simulink model "kundur_to_area_ps"  (R2018a)
settings: Solver=VariableStepDiscrete  StartTime=0.0  StopTime=10.0  RelTol=1e-3
libraries: powerlib x43, sps_avr x3, simulink x3, powerlib_meascontrol x1
settings Model: Creator=Bhaskar  LastModifiedBy=Bhaskar

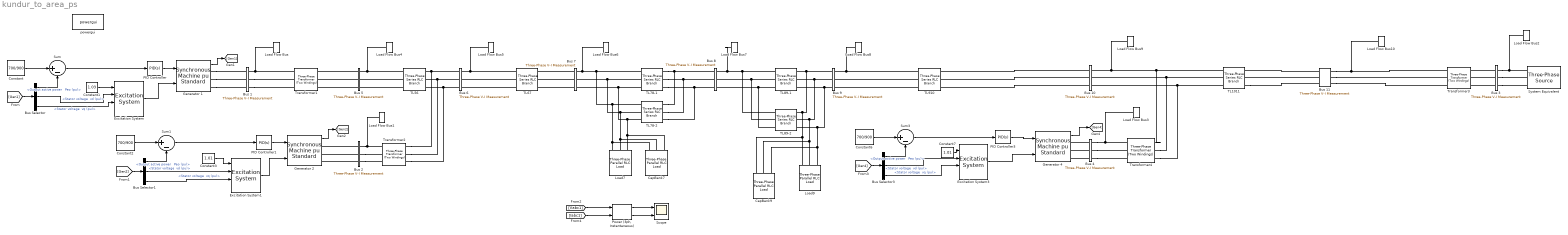
== system kundur_to_area_ps ==
  " Transformer1 " : powerlib/Elements/Three-Phase Transformer (Two Windings)  Winding1Connection=Yg  Winding2Connection=Yg  CoreType=Three single-phase transformers  SetSaturation=off  Hysteresis=off  DataFile='hysteresis'  SetInitialFlux=off  Measurements=None  UNITS=pu  NominalPower=[ 900e6 60]  Winding1=[ 20e3 0 198.944e-6 ]  Winding2="[ 230e3  0 198.944e-6]"  Rm=500  Lm=500  L0=0.5  Saturation=[ 0,0 ; 0.0024,1.2 ; 1.0,1.52 ]  InitialFluxes=[ 0.8 , -0.8 , 0.7 ]  MoreParameters=off  BreakLoop=off  DataType=off  TransfoNumber=1
  " Transformer2" : powerlib/Elements/Three-Phase Transformer (Two Windings)  Winding1Connection=Yg  Winding2Connection=Yg  CoreType=Three single-phase transformers  SetSaturation=off  Hysteresis=off  DataFile='hysteresis'  SetInitialFlux=off  Measurements=None  UNITS=pu  NominalPower=[ 900e6 60]  Winding1=[ 20e3 0 198.944e-6 ]  Winding2="[ 230e3  0 198.944e-6]"  Rm=500  Lm=500  L0=0.5  Saturation=[ 0,0 ; 0.0024,1.2 ; 1.0,1.52 ]  InitialFluxes=[ 0.8 , -0.8 , 0.7 ]  MoreParameters=off  BreakLoop=off  DataType=off  TransfoNumber=1
  " Transformer3" : powerlib/Elements/Three-Phase Transformer (Two Windings)  Winding1Connection=Yg  Winding2Connection=Yg  CoreType=Three single-phase transformers  SetSaturation=off  Hysteresis=off  DataFile='hysteresis'  SetInitialFlux=off  Measurements=None  UNITS=pu  NominalPower=[ 900e6 60]  Winding1=[ 20e3 0 198.944e-6 ]  Winding2="[ 230e3  0 198.944e-6]"  Rm=500  Lm=500  L0=0.5  Saturation=[ 0,0 ; 0.0024,1.2 ; 1.0,1.52 ]  InitialFluxes=[ 0.8 , -0.8 , 0.7 ]  MoreParameters=off  BreakLoop=off  DataType=off  TransfoNumber=1
  " Transformer4" : powerlib/Elements/Three-Phase Transformer (Two Windings)  Winding1Connection=Yg  Winding2Connection=Yg  CoreType=Three single-phase transformers  SetSaturation=off  Hysteresis=off  DataFile='hysteresis'  SetInitialFlux=off  Measurements=None  UNITS=pu  NominalPower=[ 900e6 60]  Winding1=[ 20e3 0 198.944e-6 ]  Winding2="[ 230e3  0 198.944e-6]"  Rm=500  Lm=500  L0=0.5  Saturation=[ 0,0 ; 0.0024,1.2 ; 1.0,1.52 ]  InitialFluxes=[ 0.8 , -0.8 , 0.7 ]  MoreParameters=off  BreakLoop=off  DataType=off  TransfoNumber=1
  " CapBank7" : powerlib/Elements/Three-Phase Parallel RLC Load  LConnTagsString=A|B|C  Configuration=Y (grounded)  NominalVoltage=230e3*0.8959  Vabc=[1e3 1e3 1e3]  Vabcp=[1e3 1e3 1e3]  NominalFrequency=60  UnbalancedPower=off  ActivePower=0  InductivePower=0  CapacitivePower=200e6  Pabc=[10e3 9e3 11e3]  QLabc=[100 90 110]  QCabc=[100 90 110]  Pabcp=[10e3 9e3 11e3]  QLabcp=[100 90 110]  QCabcp=[100 90 110]  Measurements=None  LoadType=constant Z
  " CapBank9" : powerlib/Elements/Three-Phase Parallel RLC Load  LConnTagsString=A|B|C  Configuration=Y (grounded)  NominalVoltage=230e3*0.9667  Vabc=[1e3 1e3 1e3]  Vabcp=[1e3 1e3 1e3]  NominalFrequency=60  UnbalancedPower=off  ActivePower=0  InductivePower=0  CapacitivePower=350e6  Pabc=[10e3 9e3 11e3]  QLabc=[100 90 110]  QCabc=[100 90 110]  Pabcp=[10e3 9e3 11e3]  QLabcp=[100 90 110]  QCabcp=[100 90 110]  Measurements=None  LoadType=constant Z
  " Load7" : powerlib/Elements/Three-Phase Parallel RLC Load  LConnTagsString=A|B|C  Configuration=Y (grounded)  NominalVoltage=230e3*0.8959  Vabc=[1e3 1e3 1e3]  Vabcp=[1e3 1e3 1e3]  NominalFrequency=60  UnbalancedPower=off  ActivePower=967e6  InductivePower=100e6  CapacitivePower=0  Pabc=[10e3 9e3 11e3]  QLabc=[100 90 110]  QCabc=[100 90 110]  Pabcp=[10e3 9e3 11e3]  QLabcp=[100 90 110]  QCabcp=[100 90 110]  Measurements=None  LoadType=constant Z
  " Load9" : powerlib/Elements/Three-Phase Parallel RLC Load  LConnTagsString=A|B|C  Configuration=Y (grounded)  NominalVoltage=230e3*0.9667  Vabc=[1e3 1e3 1e3]  Vabcp=[1e3 1e3 1e3]  NominalFrequency=60  UnbalancedPower=off  ActivePower=1767e6  InductivePower=100e6  CapacitivePower=0  Pabc=[10e3 9e3 11e3]  QLabc=[100 90 110]  QCabc=[100 90 110]  Pabcp=[10e3 9e3 11e3]  QLabcp=[100 90 110]  QCabcp=[100 90 110]  Measurements=None  LoadType=constant Z
  Bus Selector : BusSelector  OutputSignals="Output active power   Peo (pu),dq0 components.Stator voltage  vd (pu),dq0 components.Stator voltage  vq (pu)"
  Bus Selector1 : BusSelector  OutputSignals="Output active power   Peo (pu),dq0 components.Stator voltage  vd (pu),dq0 components.Stator voltage  vq (pu)"
  Bus Selector3 : BusSelector  OutputSignals="Output active power   Peo (pu),dq0 components.Stator voltage  vd (pu),dq0 components.Stator voltage  vq (pu)"
  Bus 1 : powerlib/Measurements/Three-Phase V-I Measurement  VoltageMeasurement=phase-to-ground  SetLabelV=on  LabelV=Vabc1  Vpu=off  VpuLL=off  CurrentMeasurement=yes  SetLabelI=on  LabelI=Iabc1  Ipu=off  Pbase=100e6  Vbase=500e3  OutputType=Complex  PhasorSimulation=off  PSBequivalent=0
  Bus 10 : powerlib/Measurements/Three-Phase V-I Measurement  VoltageMeasurement=phase-to-ground  SetLabelV=on  LabelV=Vabc10  Vpu=off  VpuLL=off  CurrentMeasurement=yes  SetLabelI=on  LabelI=Iabc10  Ipu=off  Pbase=100e6  Vbase=500e3  OutputType=Complex  PhasorSimulation=off  PSBequivalent=0
  Bus 11 : powerlib/Measurements/Three-Phase V-I Measurement  VoltageMeasurement=phase-to-ground  SetLabelV=on  LabelV=Vabc11  Vpu=off  VpuLL=off  CurrentMeasurement=yes  SetLabelI=on  LabelI=Iabc11  Ipu=off  Pbase=100e6  Vbase=500e3  OutputType=Complex  PhasorSimulation=off  PSBequivalent=0
  Bus 2 : powerlib/Measurements/Three-Phase V-I Measurement  VoltageMeasurement=phase-to-ground  SetLabelV=on  LabelV=Vabc2  Vpu=off  VpuLL=off  CurrentMeasurement=yes  SetLabelI=on  LabelI=Iabc2  Ipu=off  Pbase=100e6  Vbase=500e3  OutputType=Complex  PhasorSimulation=off  PSBequivalent=0
  Bus 3 : powerlib/Measurements/Three-Phase V-I Measurement  VoltageMeasurement=phase-to-ground  SetLabelV=on  LabelV=Vabc3  Vpu=off  VpuLL=off  CurrentMeasurement=yes  SetLabelI=on  LabelI=Iabc3  Ipu=off  Pbase=100e6  Vbase=500e3  OutputType=Complex  PhasorSimulation=off  PSBequivalent=0
  Bus 4 : powerlib/Measurements/Three-Phase V-I Measurement  VoltageMeasurement=phase-to-ground  SetLabelV=on  LabelV=Vabc4  Vpu=off  VpuLL=off  CurrentMeasurement=yes  SetLabelI=on  LabelI=Iabc4  Ipu=off  Pbase=100e6  Vbase=500e3  OutputType=Complex  PhasorSimulation=off  PSBequivalent=0
  Bus 5 : powerlib/Measurements/Three-Phase V-I Measurement  VoltageMeasurement=phase-to-ground  SetLabelV=on  LabelV=Vabc5  Vpu=off  VpuLL=off  CurrentMeasurement=yes  SetLabelI=on  LabelI=Iabc5  Ipu=off  Pbase=100e6  Vbase=500e3  OutputType=Complex  PhasorSimulation=off  PSBequivalent=0
  Bus 6 : powerlib/Measurements/Three-Phase V-I Measurement  VoltageMeasurement=phase-to-ground  SetLabelV=on  LabelV=Vabc6  Vpu=off  VpuLL=off  CurrentMeasurement=yes  SetLabelI=on  LabelI=Iabc6  Ipu=off  Pbase=100e6  Vbase=500e3  OutputType=Complex  PhasorSimulation=off  PSBequivalent=0
  Bus 7 : powerlib/Measurements/Three-Phase V-I Measurement  VoltageMeasurement=phase-to-ground  SetLabelV=on  LabelV=Vabc7  Vpu=off  VpuLL=off  CurrentMeasurement=yes  SetLabelI=on  LabelI=Iabc7  Ipu=off  Pbase=100e6  Vbase=500e3  OutputType=Complex  PhasorSimulation=off  PSBequivalent=0
  Bus 8 : powerlib/Measurements/Three-Phase V-I Measurement  VoltageMeasurement=phase-to-ground  SetLabelV=on  LabelV=Vabc8  Vpu=off  VpuLL=off  CurrentMeasurement=yes  SetLabelI=on  LabelI=Iabc8  Ipu=off  Pbase=100e6  Vbase=500e3  OutputType=Complex  PhasorSimulation=off  PSBequivalent=0
  Bus 9 : powerlib/Measurements/Three-Phase V-I Measurement  VoltageMeasurement=phase-to-ground  SetLabelV=on  LabelV=Vabc9  Vpu=off  VpuLL=off  CurrentMeasurement=yes  SetLabelI=on  LabelI=Iabc9  Ipu=off  Pbase=100e6  Vbase=500e3  OutputType=Complex  PhasorSimulation=off  PSBequivalent=0
  Constant : Constant  Value=700/900
  Constant1 : Constant  Value=1.03
  Constant2 : Constant  Value=700/900
  Constant3 : Constant  Value=1.01
  Constant6 : Constant  Value=700/900
  Constant7 : Constant  Value=1.01
  Excitation System : sps_avr/Excitation System  tr=0.05  reg=[ 20 0.055 ]  exc=[ 1 0 ]  tgr=[ 0 0 ]  damp=[ 0.125 1.8 ]  sat=[ 0, 0 ]  lim=[ -10 10 0 ]  v0=[0.97727 1.973]
      settings: SourceProductName=Simscape Power Systems  SourceProductBaseCode=PS
  Excitation System1 : sps_avr/Excitation System  tr=0.05  reg=[ 20 0.055 ]  exc=[ 1 0 ]  tgr=[ 0 0 ]  damp=[ 0.125 1.8 ]  sat=[ 0, 0 ]  lim=[ -10 10 0 ]  v0=[0.92904 2.0814]
      settings: SourceProductName=Simscape Power Systems  SourceProductBaseCode=PS
  Excitation System3 : sps_avr/Excitation System  tr=0.05  reg=[ 20 0.055 ]  exc=[ 1 0 ]  tgr=[ 0 0 ]  damp=[ 0.125 1.8 ]  sat=[ 0, 0 ]  lim=[ -10 10 0 ]  v0=[0.99804 1.9844]
      settings: SourceProductName=Simscape Power Systems  SourceProductBaseCode=PS
  "Generator 1 " : powerlib/Machines/Synchronous Machine pu Standard  PresetModel=No  MechanicalLoad=Mechanical power Pm  ShowDetailedParameters=on  RotorType=Round  Units=per unit standard parameters  MeasurementBus=off  NominalParameters=[900e6 20e3 60]  Reactances1=[ 1.80 0.30 0.25 1.70 0.55 0.25 0.20 ]  Reactances2=[2.24 0.17 0.12 1.02 0.13 0.08]  dAxisTimeConstants=Open-circuit  qAxisTimeConstants=Open-circuit  TimeConstants1="[ 4.4849  0.0681  0.1  ]"  TimeConstants2=[ 8.0, 0.03, 0.4, 0.05 ]  TimeConstants3="[  4.49  0.0681  0.0513  ]"  TimeConstants4=[ 8.0, 0.03, 0.3371, 0.0295 ]  TimeConstants5=[ 1.01, 0.053, 0.1 ]  TimeConstants6=[ 1.3201, 0.023, 1.0, 0.07 ]  TimeConstants7=[0.012 0.003 0.003]  TimeConstants8=[ 1.3201, 0.0231, 0.3371, 0.0295 ]  StatorResistance=0.0025  Mechanical=[6.50 0.02 1]  PolePairs=20  InitialConditions=[0 9.5032 0.823193 0.823193 0.823193 39.3665 -80.6335 159.366 1.97303]  SetSaturation=off  Saturation=[0.6404,0.7127,0.8441,0.9214,0.9956,1.082,1.19,1.316,1.457;0.7,0.7698,0.8872,0.9466,0.9969,1.046,1.1,1.151,1.201]  LoadFlowParameters=[1,0,0,0,0]  TsPowergui=0  TsBlock=-1  IterativeModel=Trapezoidal non iterative  IterativeDiscreteModel=Trapezoidal non iterative  BusType=PQ  Pref=700e6  Qref=185e6  Qmin=-inf  Qmax=inf  PLF=0  QLF=0
      settings: SourceProductName=Simscape Power Systems
  "Generator 2 " : powerlib/Machines/Synchronous Machine pu Standard  PresetModel=No  MechanicalLoad=Mechanical power Pm  ShowDetailedParameters=on  RotorType=Round  Units=per unit standard parameters  MeasurementBus=off  NominalParameters=[900e6 20e3 60]  Reactances1=[ 1.80 0.30 0.25 1.70 0.55 0.25 0.20 ]  Reactances2=[2.24 0.17 0.12 1.02 0.13 0.08]  dAxisTimeConstants=Open-circuit  qAxisTimeConstants=Open-circuit  TimeConstants1="[ 4.4849  0.0681  0.1  ]"  TimeConstants2=[ 8.0, 0.03, 0.4, 0.05 ]  TimeConstants3="[  4.49  0.0681  0.0513  ]"  TimeConstants4=[ 8.0, 0.03, 0.3371, 0.0295 ]  TimeConstants5=[ 1.01, 0.053, 0.1 ]  TimeConstants6=[ 1.3201, 0.023, 1.0, 0.07 ]  TimeConstants7=[0.012 0.003 0.003]  TimeConstants8=[ 1.3201, 0.0231, 0.3371, 0.0295 ]  StatorResistance=0.0025  Mechanical=[6.50 0.02 1]  PolePairs=20  InitialConditions=[0 -1.3462 0.883102 0.883102 0.883102 24.8213 -95.1787 144.821 2.08141]  SetSaturation=off  Saturation=[0.6404,0.7127,0.8441,0.9214,0.9956,1.082,1.19,1.316,1.457;0.7,0.7698,0.8872,0.9466,0.9969,1.046,1.1,1.151,1.201]  LoadFlowParameters=[1,0,0,0,0]  TsPowergui=0  TsBlock=-1  IterativeModel=Trapezoidal non iterative  IterativeDiscreteModel=Trapezoidal non iterative  BusType=PQ  Pref=700e6  Qref=235e6  Qmin=-inf  Qmax=inf  PLF=0  QLF=0
      settings: SourceProductName=Simscape Power Systems
  Generator 4 : powerlib/Machines/Synchronous Machine pu Standard  PresetModel=No  MechanicalLoad=Mechanical power Pm  ShowDetailedParameters=on  RotorType=Round  Units=per unit standard parameters  MeasurementBus=off  NominalParameters=[900e6 20e3 60]  Reactances1=[ 1.80 0.30 0.25 1.70 0.55 0.25 0.20 ]  Reactances2=[2.24 0.17 0.12 1.02 0.13 0.08]  dAxisTimeConstants=Open-circuit  qAxisTimeConstants=Open-circuit  TimeConstants1="[ 4.4849  0.0681  0.1  ]"  TimeConstants2=[ 8.0, 0.03, 0.4, 0.05 ]  TimeConstants3="[  4.49  0.0681  0.0513  ]"  TimeConstants4=[ 8.0, 0.03, 0.3371, 0.0295 ]  TimeConstants5=[ 1.01, 0.053, 0.1 ]  TimeConstants6=[ 1.3201, 0.023, 1.0, 0.07 ]  TimeConstants7=[0.012 0.003 0.003]  TimeConstants8=[ 1.3201, 0.0231, 0.3371, 0.0295 ]  StatorResistance=0.0025  Mechanical=[6.175 0.02 1]  PolePairs=20  InitialConditions=[0 -52.16 0.811101 0.811101 0.811101 -22.028 -142.028 97.972 1.98441]  SetSaturation=off  Saturation=[0.6404,0.7127,0.8441,0.9214,0.9956,1.082,1.19,1.316,1.457;0.7,0.7698,0.8872,0.9466,0.9969,1.046,1.1,1.151,1.201]  LoadFlowParameters=[1,0,0,0,0]  TsPowergui=0  TsBlock=-1  IterativeModel=Trapezoidal non iterative  IterativeDiscreteModel=Trapezoidal non iterative  BusType=PQ  Pref=700e6  Qref=202e6  Qmin=-inf  Qmax=inf  PLF=0  QLF=0
      settings: SourceProductName=Simscape Power Systems
  Load Flow Bus : powerlib/Measurements/Load Flow Bus  LConnTagsString=a  Phases=single  Connectors=on one side  ID=BUS_1  Vbase=20e3  Vref=1  Vangle=0  VLF=0.9773  VLFb=1  VLFc=1  angleLF=54.17  angleLFb=0  angleLFc=0
      settings: SourceProductName=Simscape Power Systems
  Load Flow Bus1 : powerlib/Measurements/Load Flow Bus  LConnTagsString=a  Phases=single  Connectors=on one side  ID=BUS_2  Vbase=20e3  Vref=1  Vangle=0  VLF=0.929  VLFb=1  VLFc=1  angleLF=43.38  angleLFb=0  angleLFc=0
      settings: SourceProductName=Simscape Power Systems
  Load Flow Bus10 : powerlib/Measurements/Load Flow Bus  LConnTagsString=a  Phases=single  Connectors=on one side  ID=BUS_11  Vbase=230e3  Vref=1  Vangle=0  VLF=1.03  VLFb=1  VLFc=1  angleLF=-0.01044  angleLFb=0  angleLFc=0
      settings: SourceProductName=Simscape Power Systems
  Load Flow Bus2 : powerlib/Measurements/Load Flow Bus  LConnTagsString=a  Phases=single  Connectors=on one side  ID=BUS_3  Vbase=20e3  Vref=1.03  Vangle=0  VLF=1.03  VLFb=1  VLFc=1  angleLF=0  angleLFb=0  angleLFc=0
      settings: SourceProductName=Simscape Power Systems
  Load Flow Bus3 : powerlib/Measurements/Load Flow Bus  LConnTagsString=a  Phases=single  Connectors=on one side  ID=BUS_4  Vbase=20e3  Vref=1  Vangle=0  VLF=0.998  VLFb=1  VLFc=1  angleLF=-5.931  angleLFb=0  angleLFc=0
      settings: SourceProductName=Simscape Power Systems
  Load Flow Bus4 : powerlib/Measurements/Load Flow Bus  LConnTagsString=a  Phases=single  Connectors=on one side  ID=BUS_5  Vbase=230e3  Vref=1  Vangle=0  VLF=0.9772  VLFb=1  VLFc=1  angleLF=54.15  angleLFb=0  angleLFc=0
      settings: SourceProductName=Simscape Power Systems
  Load Flow Bus5 : powerlib/Measurements/Load Flow Bus  LConnTagsString=a  Phases=single  Connectors=on one side  ID=BUS_6  Vbase=230e3  Vref=1  Vangle=0  VLF=0.9289  VLFb=1  VLFc=1  angleLF=43.36  angleLFb=0  angleLFc=0
      settings: SourceProductName=Simscape Power Systems
  Load Flow Bus6 : powerlib/Measurements/Load Flow Bus  LConnTagsString=a  Phases=single  Connectors=on one side  ID=BUS_7  Vbase=230e3  Vref=1  Vangle=0  VLF=0.8959  VLFb=1  VLFc=1  angleLF=33.99  angleLFb=0  angleLFc=0
      settings: SourceProductName=Simscape Power Systems
  Load Flow Bus7 : powerlib/Measurements/Load Flow Bus  LConnTagsString=a  Phases=single  Connectors=on one side  ID=BUS_8  Vbase=230e3  Vref=1  Vangle=0  VLF=0.8557  VLFb=1  VLFc=1  angleLF=9.8  angleLFb=0  angleLFc=0
      settings: SourceProductName=Simscape Power Systems
  Load Flow Bus8 : powerlib/Measurements/Load Flow Bus  LConnTagsString=a  Phases=single  Connectors=on one side  ID=BUS_9  Vbase=230e3  Vref=1  Vangle=0  VLF=0.9667  VLFb=1  VLFc=1  angleLF=-12.52  angleLFb=0  angleLFc=0
      settings: SourceProductName=Simscape Power Systems
  Load Flow Bus9 : powerlib/Measurements/Load Flow Bus  LConnTagsString=a  Phases=single  Connectors=on one side  ID=BUS_10  Vbase=230e3  Vref=1  Vangle=0  VLF=0.998  VLFb=1  VLFc=1  angleLF=-5.949  angleLFb=0  angleLFc=0
      settings: SourceProductName=Simscape Power Systems
  PID Controller : simulink/Continuous/PID Controller  Controller=PID  TimeDomain=Continuous-time  SampleTime=-1  IntegratorMethod=Forward Euler  FilterMethod=Forward Euler  Form=Parallel  UseFilter=on  ControllerParametersSource=internal  P=1  I=2  D=0.2  N=100  InitialConditionSource=internal  InitialConditionForIntegrator=0  InitialConditionForFilter=0  ExternalReset=none  LimitOutput=on  UpperSaturationLimit=0.99  LowerSaturationLimit=0.50  LinearizeAsGain=on  AntiWindupMode=none  Kb=1  TrackingMode=off  Kt=1  PParamMin=[]  PParamMax=[]  IParamMin=[]  IParamMax=[]  DParamMin=[]  DParamMax=[]  NParamMin=[]  NParamMax=[]  KbParamMin=[]  KbParamMax=[]  KtParamMin=[]  KtParamMax=[]  POutMin=[]  POutMax=[]  IOutMin=[]  IOutMax=[]  DOutMin=[]  DOutMax=[]  NOutMin=[]  NOutMax=[]  KbOutMin=[]  KbOutMax=[]  KtOutMin=[]  KtOutMax=[]  IntegratorOutMin=[]  IntegratorOutMax=[]  FilterOutMin=[]  FilterOutMax=[]  SumOutMin=[]  SumOutMax=[]  SumI1OutMin=[]  SumI1OutMax=[]  SumI2OutMin=[]  SumI2OutMax=[]  SumI3OutMin=[]  SumI3OutMax=[]  SumDOutMin=[]  SumDOutMax=[]  SaturationOutMin=[]  SaturationOutMax=[]  IntegratorContinuousStateAttributes=''  IntegratorStateMustResolveToSignalObject=off  IntegratorRTWStateStorageClass=Auto  FilterContinuousStateAttributes=''  FilterStateMustResolveToSignalObject=off  FilterRTWStateStorageClass=Auto  DifferentiatorICPrevScaledInput=0  DifferentiatorOutMin=[]  DifferentiatorOutMax=[]  FilterDiffOutCoefMin=[]  FilterDiffOutCoefMax=[]  SumDenOutMin=[]  SumDenOutMax=[]  SumNumOutMin=[]  SumNumOutMax=[]  ReciprocalOutMin=[]  ReciprocalOutMax=[]  DivideOutMin=[]  DivideOutMax=[]  TunerSelectOption=Transfer Function Based (PID Tuner App)
  PID Controller1 : simulink/Continuous/PID Controller  Controller=PID  TimeDomain=Continuous-time  SampleTime=-1  IntegratorMethod=Forward Euler  FilterMethod=Forward Euler  Form=Parallel  UseFilter=on  ControllerParametersSource=internal  P=1  I=2  D=0.2  N=100  InitialConditionSource=internal  InitialConditionForIntegrator=0  InitialConditionForFilter=0  ExternalReset=none  LimitOutput=on  UpperSaturationLimit=0.99  LowerSaturationLimit=0.50  LinearizeAsGain=on  AntiWindupMode=none  Kb=1  TrackingMode=off  Kt=1  PParamMin=[]  PParamMax=[]  IParamMin=[]  IParamMax=[]  DParamMin=[]  DParamMax=[]  NParamMin=[]  NParamMax=[]  KbParamMin=[]  KbParamMax=[]  KtParamMin=[]  KtParamMax=[]  POutMin=[]  POutMax=[]  IOutMin=[]  IOutMax=[]  DOutMin=[]  DOutMax=[]  NOutMin=[]  NOutMax=[]  KbOutMin=[]  KbOutMax=[]  KtOutMin=[]  KtOutMax=[]  IntegratorOutMin=[]  IntegratorOutMax=[]  FilterOutMin=[]  FilterOutMax=[]  SumOutMin=[]  SumOutMax=[]  SumI1OutMin=[]  SumI1OutMax=[]  SumI2OutMin=[]  SumI2OutMax=[]  SumI3OutMin=[]  SumI3OutMax=[]  SumDOutMin=[]  SumDOutMax=[]  SaturationOutMin=[]  SaturationOutMax=[]  IntegratorContinuousStateAttributes=''  IntegratorStateMustResolveToSignalObject=off  IntegratorRTWStateStorageClass=Auto  FilterContinuousStateAttributes=''  FilterStateMustResolveToSignalObject=off  FilterRTWStateStorageClass=Auto  DifferentiatorICPrevScaledInput=0  DifferentiatorOutMin=[]  DifferentiatorOutMax=[]  FilterDiffOutCoefMin=[]  FilterDiffOutCoefMax=[]  SumDenOutMin=[]  SumDenOutMax=[]  SumNumOutMin=[]  SumNumOutMax=[]  ReciprocalOutMin=[]  ReciprocalOutMax=[]  DivideOutMin=[]  DivideOutMax=[]  TunerSelectOption=Transfer Function Based (PID Tuner App)
  PID Controller3 : simulink/Continuous/PID Controller  Controller=PID  TimeDomain=Continuous-time  SampleTime=-1  IntegratorMethod=Forward Euler  FilterMethod=Forward Euler  Form=Parallel  UseFilter=on  ControllerParametersSource=internal  P=1  I=2  D=0.2  N=100  InitialConditionSource=internal  InitialConditionForIntegrator=0  InitialConditionForFilter=0  ExternalReset=none  LimitOutput=on  UpperSaturationLimit=0.99  LowerSaturationLimit=0.50  LinearizeAsGain=on  AntiWindupMode=none  Kb=1  TrackingMode=off  Kt=1  PParamMin=[]  PParamMax=[]  IParamMin=[]  IParamMax=[]  DParamMin=[]  DParamMax=[]  NParamMin=[]  NParamMax=[]  KbParamMin=[]  KbParamMax=[]  KtParamMin=[]  KtParamMax=[]  POutMin=[]  POutMax=[]  IOutMin=[]  IOutMax=[]  DOutMin=[]  DOutMax=[]  NOutMin=[]  NOutMax=[]  KbOutMin=[]  KbOutMax=[]  KtOutMin=[]  KtOutMax=[]  IntegratorOutMin=[]  IntegratorOutMax=[]  FilterOutMin=[]  FilterOutMax=[]  SumOutMin=[]  SumOutMax=[]  SumI1OutMin=[]  SumI1OutMax=[]  SumI2OutMin=[]  SumI2OutMax=[]  SumI3OutMin=[]  SumI3OutMax=[]  SumDOutMin=[]  SumDOutMax=[]  SaturationOutMin=[]  SaturationOutMax=[]  IntegratorContinuousStateAttributes=''  IntegratorStateMustResolveToSignalObject=off  IntegratorRTWStateStorageClass=Auto  FilterContinuousStateAttributes=''  FilterStateMustResolveToSignalObject=off  FilterRTWStateStorageClass=Auto  DifferentiatorICPrevScaledInput=0  DifferentiatorOutMin=[]  DifferentiatorOutMax=[]  FilterDiffOutCoefMin=[]  FilterDiffOutCoefMax=[]  SumDenOutMin=[]  SumDenOutMax=[]  SumNumOutMin=[]  SumNumOutMax=[]  ReciprocalOutMin=[]  ReciprocalOutMax=[]  DivideOutMin=[]  DivideOutMax=[]  TunerSelectOption=Transfer Function Based (PID Tuner App)
  "Power (3ph, Instantaneous)" : powerlib_meascontrol/Measurements/Power (3ph, Instantaneous)
      settings: SourceProductName=Simscape Power Systems
  Scope : Scope  NumInputPorts=2
  Sum : Sum  Inputs=|+-
  Sum1 : Sum  Inputs=|+-
  Sum3 : Sum  Inputs=|+-
  System Equivalent : powerlib/Electrical Sources/Three-Phase Source  InternalConnection=Yg  VoltagePhases=off  Voltage=(20000)*1.03  PhaseAngle=0  Voltage_phases=[25e3 25e3 25e3]/sqrt(3)  PhaseAngles_phases=[0 -120 +120]  Frequency=60  NonIdealSource=off  SpecifyImpedance=off  Resistance=0.8929  Inductance=16.58e-3  ShortCircuitLevel=100e6  BaseVoltage=25e3  XRratio=7  BusType=swing  Pref=10e3  Qref=0  Prefabc=[10e3, 10e3, 10e3]  Qrefabc=[0, 0, 0]  Qmin=-inf  Qmax=inf
  TL1011 : powerlib/Elements/Three-Phase Series RLC Branch  LConnTagsString=A|B|C  RConnTagsString=A|B|C  BranchType=RL  Resistance=1.3225  Inductance=3.508e-2  Capacitance=1e-6  Measurements=None
  "TL56 " : powerlib/Elements/Three-Phase Series RLC Branch  LConnTagsString=A|B|C  RConnTagsString=A|B|C  BranchType=RL  Resistance=1.3225  Inductance=3.508e-2  Capacitance=1e-6  Measurements=None
  TL67 : powerlib/Elements/Three-Phase Series RLC Branch  LConnTagsString=A|B|C  RConnTagsString=A|B|C  BranchType=RL  Resistance=0.529  Inductance=1.403e-2  Capacitance=1e-6  Measurements=None
  TL78-1 : powerlib/Elements/Three-Phase Series RLC Branch  LConnTagsString=A|B|C  RConnTagsString=A|B|C  BranchType=RL  Resistance=5.819  Inductance=1.544e-1  Capacitance=1e-6  Measurements=None
  TL78-2 : powerlib/Elements/Three-Phase Series RLC Branch  LConnTagsString=A|B|C  RConnTagsString=A|B|C  BranchType=RL  Resistance=5.819  Inductance=1.544e-1  Capacitance=1e-6  Measurements=None
  TL89-1 : powerlib/Elements/Three-Phase Series RLC Branch  LConnTagsString=A|B|C  RConnTagsString=A|B|C  BranchType=RL  Resistance=5.819  Inductance=1.544e-1  Capacitance=1e-6  Measurements=None
  TL89-2 : powerlib/Elements/Three-Phase Series RLC Branch  LConnTagsString=A|B|C  RConnTagsString=A|B|C  BranchType=RL  Resistance=5.819  Inductance=1.544e-1  Capacitance=1e-6  Measurements=None
  TL910 : powerlib/Elements/Three-Phase Series RLC Branch  LConnTagsString=A|B|C  RConnTagsString=A|B|C  BranchType=RL  Resistance=0.529  Inductance=1.403e-2  Capacitance=1e-6  Measurements=None
  powergui : powerlib/powergui  Priority=1  SimulationMode=Discrete  SampleTime=500e-6  frequency=60  Iterations=1000  frequencyindice=60  Pbase=100e6  ErrMax=0.0001  UnitsV=kV  UnitsW=MW  buscounter=0  FunctionMessages=off  echomessages=off  EnableUseOfTLC=off  CurrentSourceSwitches=off  DisableSnubberDevices=off  DisableRonSwitches=off  DisableVfSwitches=off  DisplayEquations=off  SolverType=Tustin/Backward Euler (TBE)  Interpol=off  ExternalGateDelay=off  methode=off  Ts=100  x0status=blocks  SPID=on  SwTol=0  HookPort=off  RestoreLinks=warning  ResistiveCurrentMeasurement=off  Frange=[0:2:500]  Ylog=off  Xlog=on  ShowGrid=off  save=off  variable=ZData  structure=0  ZoomFFT=off  StartTime=0.0  cycles=1  DisplayStyle=1  fundamental=60  FreqAxis=off  MaxFrequency=1000  frequencyindicesteady=1  RmsSteady=1  display=off
  wires:
  "Generator 1 "/1 -> [Gen1]
  [Gen1] -> Bus Selector/1
  PID Controller/1 -> "Generator 1 "/1
  Sum/1 -> PID Controller/1
  Constant/1 -> Sum/1
  Bus Selector/1 -> Sum/2  "<Output active power   Peo (pu)>"
  Constant1/1 -> Excitation System/1
  Bus Selector/2 -> Excitation System/2  "<Stator voltage  vd (pu)>"
  Bus Selector/3 -> Excitation System/3  "<Stator voltage  vq (pu)>"
  Bus Selector1/3 -> Excitation System1/3  "<Stator voltage  vq (pu)>"
  Bus Selector1/2 -> Excitation System1/2  "<Stator voltage  vd (pu)>"
  Constant3/1 -> Excitation System1/1
  Bus Selector1/1 -> Sum1/2  "<Output active power   Peo (pu)>"
  Constant2/1 -> Sum1/1
  Sum1/1 -> PID Controller1/1
  [Gen2] -> Bus Selector1/1
  Excitation System/1 -> "Generator 1 "/2
  Excitation System1/1 -> "Generator 2 "/2
  PID Controller1/1 -> "Generator 2 "/1
  "Generator 2 "/1 -> [Gen2]
  Constant7/1 -> Excitation System3/1
  Bus Selector3/1 -> Sum3/2  "<Output active power   Peo (pu)>"
  Bus Selector3/2 -> Excitation System3/2  "<Stator voltage  vd (pu)>"
  [Gen4] -> Bus Selector3/1
  Sum3/1 -> PID Controller3/1
  Generator 4/1 -> [Gen4]
  PID Controller3/1 -> Generator 4/1
  Constant6/1 -> Sum3/1
  Bus Selector3/3 -> Excitation System3/3  "<Stator voltage  vq (pu)>"
  Excitation System3/1 -> Generator 4/2
  [Vabc1] -> "Power (3ph, Instantaneous)"/1
  [Iabc1] -> "Power (3ph, Instantaneous)"/2
  "Power (3ph, Instantaneous)"/1 -> Scope/1
  "Power (3ph, Instantaneous)"/2 -> Scope/2
  connections:
  Bus 1/RConn1 -- Load Flow Bus/LConn1 -- " Transformer1 "/LConn1
  Bus 1/RConn2 -- " Transformer1 "/LConn2
  Bus 1/RConn3 -- " Transformer1 "/LConn3
  "Generator 1 "/RConn1 -- Bus 1/LConn1
  "Generator 1 "/RConn2 -- Bus 1/LConn2
  "Generator 1 "/RConn3 -- Bus 1/LConn3
  Bus 5/LConn1 -- " Transformer1 "/RConn1
  Bus 5/LConn2 -- " Transformer1 "/RConn2
  Bus 5/LConn3 -- " Transformer1 "/RConn3
  "TL56 "/LConn1 -- Load Flow Bus4/LConn1 -- Bus 5/RConn1
  "TL56 "/LConn2 -- Bus 5/RConn2
  "TL56 "/LConn3 -- Bus 5/RConn3
  Bus 6/LConn3 -- " Transformer2"/RConn3 -- "TL56 "/RConn3
  Bus 6/LConn2 -- " Transformer2"/RConn2 -- "TL56 "/RConn2
  Bus 6/LConn1 -- " Transformer2"/RConn1 -- "TL56 "/RConn1
  TL67/LConn1 -- Load Flow Bus5/LConn1 -- Bus 6/RConn1
  TL67/LConn2 -- Bus 6/RConn2
  TL67/LConn3 -- Bus 6/RConn3
  Bus 7/LConn3 -- TL67/RConn3
  Bus 7/LConn2 -- TL67/RConn2
  Bus 7/LConn1 -- TL67/RConn1
  TL78-1/LConn1 -- " CapBank7"/LConn1 -- " Load7"/LConn1 -- TL78-2/LConn1 -- Load Flow Bus6/LConn1 -- Bus 7/RConn1
  TL78-1/LConn2 -- " CapBank7"/LConn2 -- " Load7"/LConn2 -- TL78-2/LConn2 -- Bus 7/RConn2
  TL78-1/LConn3 -- " CapBank7"/LConn3 -- " Load7"/LConn3 -- TL78-2/LConn3 -- Bus 7/RConn3
  TL78-1/RConn1 -- TL78-2/RConn1 -- Bus 8/LConn1
  TL78-1/RConn2 -- TL78-2/RConn2 -- Bus 8/LConn2
  TL78-1/RConn3 -- TL78-2/RConn3 -- Bus 8/LConn3
  TL89-1/LConn1 -- TL89-2/LConn1 -- Load Flow Bus7/LConn1 -- Bus 8/RConn1
  TL89-1/LConn2 -- TL89-2/LConn2 -- Bus 8/RConn2
  TL89-1/LConn3 -- TL89-2/LConn3 -- Bus 8/RConn3
  Bus 9/LConn1 -- " CapBank9"/LConn1 -- " Load9"/LConn1 -- TL89-2/RConn1 -- TL89-1/RConn1
  Bus 9/LConn2 -- " CapBank9"/LConn2 -- " Load9"/LConn2 -- TL89-2/RConn2 -- TL89-1/RConn2
  Bus 9/LConn3 -- " CapBank9"/LConn3 -- " Load9"/LConn3 -- TL89-2/RConn3 -- TL89-1/RConn3
  TL910/LConn1 -- Load Flow Bus8/LConn1 -- Bus 9/RConn1
  TL910/LConn2 -- Bus 9/RConn2
  TL910/LConn3 -- Bus 9/RConn3
  Bus 10/LConn3 -- TL910/RConn3
  Bus 10/LConn2 -- TL910/RConn2
  Bus 10/LConn1 -- TL910/RConn1
  TL1011/LConn1 -- " Transformer4"/RConn1 -- Load Flow Bus9/LConn1 -- Bus 10/RConn1
  TL1011/LConn2 -- " Transformer4"/RConn2 -- Bus 10/RConn2
  TL1011/LConn3 -- " Transformer4"/RConn3 -- Bus 10/RConn3
  Bus 3/LConn3 -- " Transformer3"/LConn3
  Bus 3/LConn2 -- " Transformer3"/LConn2
  Bus 3/LConn1 -- " Transformer3"/LConn1
  Bus 3/RConn1 -- Load Flow Bus2/LConn1 -- System Equivalent/RConn1
  Bus 3/RConn2 -- System Equivalent/RConn2
  Bus 3/RConn3 -- System Equivalent/RConn3
  Bus 2/LConn1 -- "Generator 2 "/RConn1
  Bus 2/LConn2 -- "Generator 2 "/RConn2
  Bus 2/LConn3 -- "Generator 2 "/RConn3
  Bus 2/RConn1 -- Load Flow Bus1/LConn1 -- " Transformer2"/LConn1
  Bus 2/RConn2 -- " Transformer2"/LConn2
  Bus 2/RConn3 -- " Transformer2"/LConn3
  Bus 11/LConn1 -- TL1011/RConn1
  Bus 11/LConn2 -- TL1011/RConn2
  Bus 11/RConn3 -- " Transformer3"/RConn3
  Bus 11/RConn2 -- " Transformer3"/RConn2
  Bus 11/RConn1 -- Load Flow Bus10/LConn1 -- " Transformer3"/RConn1
  Bus 4/LConn1 -- Generator 4/RConn1
  Bus 4/LConn2 -- Generator 4/RConn2
  Bus 4/LConn3 -- Generator 4/RConn3
  Bus 4/RConn3 -- " Transformer4"/LConn3
  Bus 4/RConn2 -- " Transformer4"/LConn2
  Bus 4/RConn1 -- Load Flow Bus3/LConn1 -- " Transformer4"/LConn1
  TL1011/RConn3 -- Bus 11/LConn3
